simulink library "ilcUpdateLaw_cl"  (R2022a)
settings: Solver=VariableStepAuto  StartTime=0.0  StopTime=10.0  RelTol=1e-3
undefined symbols (not defined in the file or in its folder): enableVec, lrn, trstRgn
settings Model: Creator=mcobb  LastModifiedBy=lhill8
settings SolverCC: AlgebraicLoopSolver=TrustRegion
settings DebuggingCC: UnconnectedInputMsg=warning  UnconnectedOutputMsg=warning  UnconnectedLineMsg=warning  SFMachineParentedDataDiag=warning  ArithmeticOperatorsInVariantConditions=warning
settings SFSimCC: CustomCodeUndefinedFunction=UseInterfaceOnly

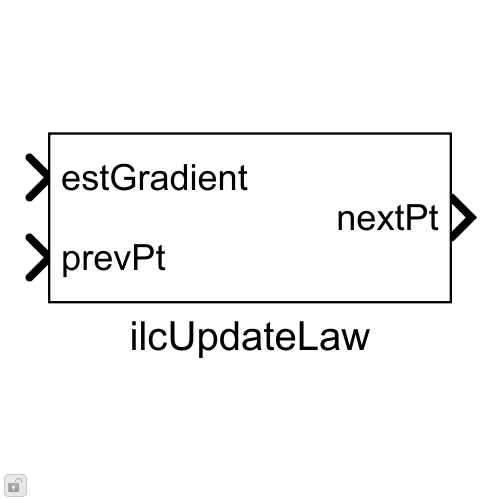
[thumbnail: Simulink's stored preview of the top-level diagram]
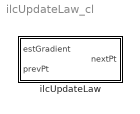
== system ilcUpdateLaw_cl ==
  ilcUpdateLaw : Subsystem  mask{lrn=lrn, trstRgn=trstRgn, amp=0}
      mask prompts: lrn "Gradient Based Learning Gain"; trstRgn "Trust Region Dimensions"; amp "White Noise Amplitude"

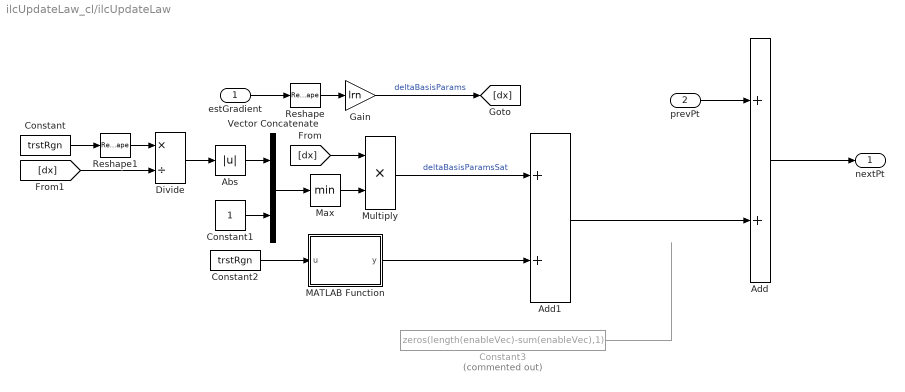
== system ilcUpdateLaw_cl/ilcUpdateLaw ==
  estGradient : Inport
  prevPt : Inport  Port=2
  Abs : Abs  SaturateOnIntegerOverflow=off
  Add : Sum
  Add1 : Sum
  Constant : Constant  Value=trstRgn
  Constant1 : Constant
  Constant2 : Constant  Value=trstRgn
  Constant3 : Constant  Commented=on  Value=zeros(length(enableVec)-sum(enableVec),1)
  Divide : Product  Inputs=*/
  Gain : Gain  Gain=lrn
  MATLAB Function : MATLAB Function  TreatAsAtomicUnit=on
  Max : MinMax
  Multiply : Product
  Reshape : Reshape  OutputDimensionality=Column vector (2-D)
  Reshape1 : Reshape  OutputDimensionality=Column vector (2-D)
  Vector Concatenate : Concatenate
  nextPt : Outport  VectorParamsAs1DForOutWhenUnconnected=off
  wires:
  Constant2/1 -> MATLAB Function/1(u)
  Abs/1 -> Vector Concatenate/1
  Vector Concatenate/1 -> Max/1
  Constant1/1 -> Vector Concatenate/2
  Max/1 -> Multiply/2
  Gain/1 -> [dx]  "deltaBasisParams"
  Add/1 -> nextPt/1
  MATLAB Function/1(y) -> Add1/2
  Reshape1/1 -> Divide/1
  Constant/1 -> Reshape1/1
  [dx] -> Divide/2
  Divide/1 -> Abs/1
  Reshape/1 -> Gain/1
  [dx] -> Multiply/1
  Multiply/1 -> Add1/1  "deltaBasisParamsSat"
  estGradient/1 -> Reshape/1
  prevPt/1 -> Add/1
  Constant3/1 -> ?
  Add1/1 -> Add/2

== matlab function ilcUpdateLaw_cl/ilcUpdateLaw/MATLAB Function ==
  data: y output; amp parameter; u input
function y = fcn(amp, u)
y = amp(:).*(2*rand([numel(u) 1])-1);
